simulink model "T3_2"  (R2022b)
settings: Solver=VariableStepAuto  StartTime=0.0  StopTime=10.0  RelTol=1e-3
InitFcn:
  | % Parámetros del sistema
  | 
  | L=1E-3; R=10; J=0.001; B=0.3; k_t=1; k_b=1; n=30;
  | N=30; M=10; b=2; k=2;
  | 
  | 
  | % Matrices
  | dospienecuadrada = (2*pi*N)^2;
  | denominador = (J*(dospienecuadrada)+(n^2)*M);
  | A = [0, 0, n/(2*pi*N); 0, -R/L, -k_b/L; -(n*k*2*pi*N)/denominador, (k_t*dospienecuadrada)/denominador, -((B*dospienecuadrada)+((n^2)*b))/denominador];
  | B = [0; 1/L; 0];
  | C = eye(3);
  | 
  | T = 10E-3;
  | Ad = eye(3)+T*A;
  | Bd = T*B;
  | Cd = C;
  | 
  | k1 = 0.5;
  | k2 = 0.5;
  | k3 =0.5;
settings Model: Creator=garci  LastModifiedBy=garci

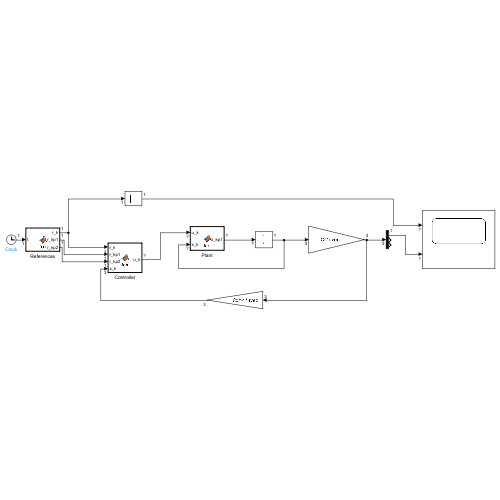
[thumbnail: Simulink's stored preview of the top-level diagram]
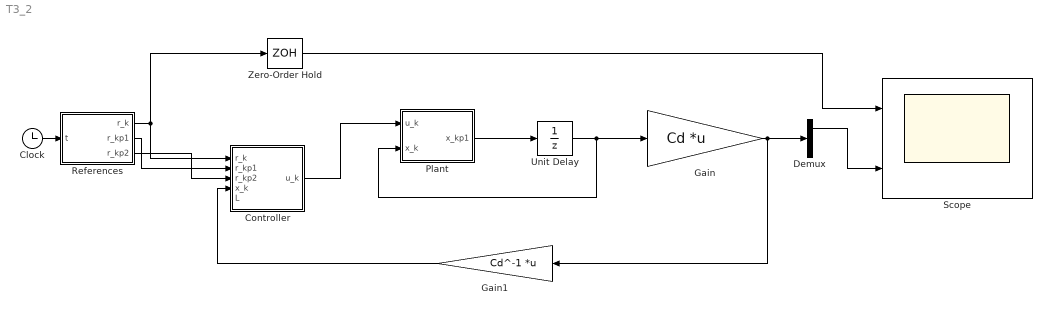
== system T3_2 ==
  Clock : Clock
  Controller : MATLAB Function  TreatAsAtomicUnit=on
  Demux : Demux  Outputs=3
  Gain : Gain  Gain=Cd  Multiplication=Matrix(K*u) (u vector)
  Gain1 : Gain  Gain=Cd^-1  Multiplication=Matrix(K*u) (u vector)
  Plant : MATLAB Function  TreatAsAtomicUnit=on
  References : MATLAB Function  TreatAsAtomicUnit=on
  Scope : Scope  NumInputPorts=2
  Unit Delay : UnitDelay  SampleTime=T  HasFrameUpgradeWarning=on
  Zero-Order Hold : ZeroOrderHold  SampleTime=T
  wires:
  Clock/1 -> References/1(t)
  References/1(r_k) -> Controller/1(r_k), Zero-Order Hold/1
  Gain/1 -> Gain1/1, Demux/1
  Zero-Order Hold/1 -> Scope/1
  Unit Delay/1 -> Plant/2(x_k), Gain/1
  Plant/1(x_kp1) -> Unit Delay/1
  Gain1/1 -> Controller/4(x_k)
  Controller/1(u_k) -> Plant/1(u_k)
  References/2(r_kp1) -> Controller/2(r_kp1)
  Demux/1 -> Scope/2
  References/3(r_kp2) -> Controller/3(r_kp2)

== matlab function T3_2/Controller ==
  data: u_k output; r_k input; r_kp1 input; r_kp2 input; x_k input; Ad parameter; Bd parameter; Cd parameter; N parameter; n parameter; k1 parameter; k2 parameter; k3 parameter; T parameter; denominador parameter; k_t parameter; L input
function u_k = fcn(r_k, r_kp1, r_kp2, x_k, Ad, Bd, Cd, N, n, k1, k2, k3, T, denominador, k_t,L)

delta = denominador;
%bloque 1
e1_k = r_k - Cd(1,:) * x_k;
x1_kp1 = x_k(1,:) + (T*(n/(2*pi*N)))* x_k(3,:);
e1_kp1 = r_kp1 - x1_kp1;
x3_ref = (r_kp1 - x_k(1,:) - k1*e1_k) * ((2*pi*N)/(n*T)); 
x3_refp1 = (r_kp2 - x1_kp1 -k1*e1_kp1) * ((2*pi*N)/(n*T));

%bloque 2


x3_kp1 = Ad(3,1)* x_k(1,:) + Ad(3,2)* x_k(2,:) + Ad(3,3)* x_k(3,:);
e2_k = x3_ref - x_k(3,:);


e2_kp1 = x3_refp1 - x3_kp1;

x2ref_k = (x3_refp1 - Ad(3,1)* x_k(1,:) - Ad(3,3)* x_k(3,:) - k2*e2_k) / ((T*k_t*(2*pi*N)^2)/(delta));
x3_refp2 =1;
x2ref_kp1 = x3_refp2- Ad(1,:)*x_k;

x1_kp2 = x_k(1,:) + (T*(n/(2*pi*N)))* x_k(3,:) + x3_kp1;

%bloque 3
e3_k = x2ref_k - x_k(2,:);
e3_kp1 = x2ref_kp1 - Ad(2,:)*-x_k;
u_k = (e3_kp1 - k3*e3_k) / (L/T);

== matlab function T3_2/References ==
  data: t input; r_k output; r_kp1 output; r_kp2 output
function [r_k,r_kp1, r_kp2] = fcn(t)

r_k = 2*sin(t);
r_kp1 = 2*sin(t+1);
r_kp2 = 2*sin(t+2);

== matlab function T3_2/Plant ==
  data: u_k input; x_kp1 output; x_k input; Bd parameter; Ad parameter
function x_kp1 = fcn(u_k, x_k, Bd, Ad)

x_kp1 = Ad*x_k + Bd*u_k;
